simulink model "MotorXploer"  (R2025a)
settings: Solver=FixedStepAuto  StartTime=0.0  StopTime=inf  FixedStep=0.001  RelTol=1e-3
undefined symbols (not defined in the file): Blocking, LF, Non
libraries: amg_usbconverter_n_connect_lib x3, dspstat3 x2, simulink x2, dspfdesign x1, waijung_addon_module x1
settings Model: Creator=beamk  LastModifiedBy=nitic

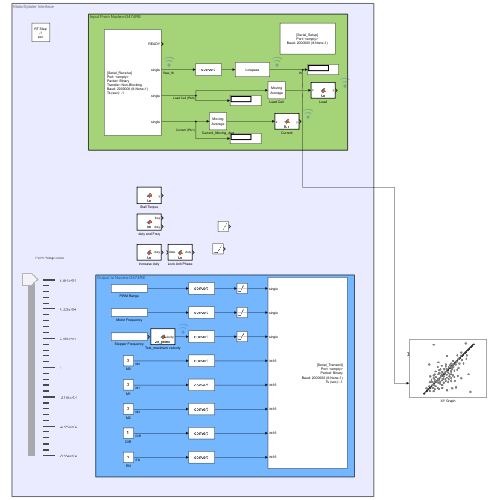
[thumbnail: Simulink's stored preview of the top-level diagram]
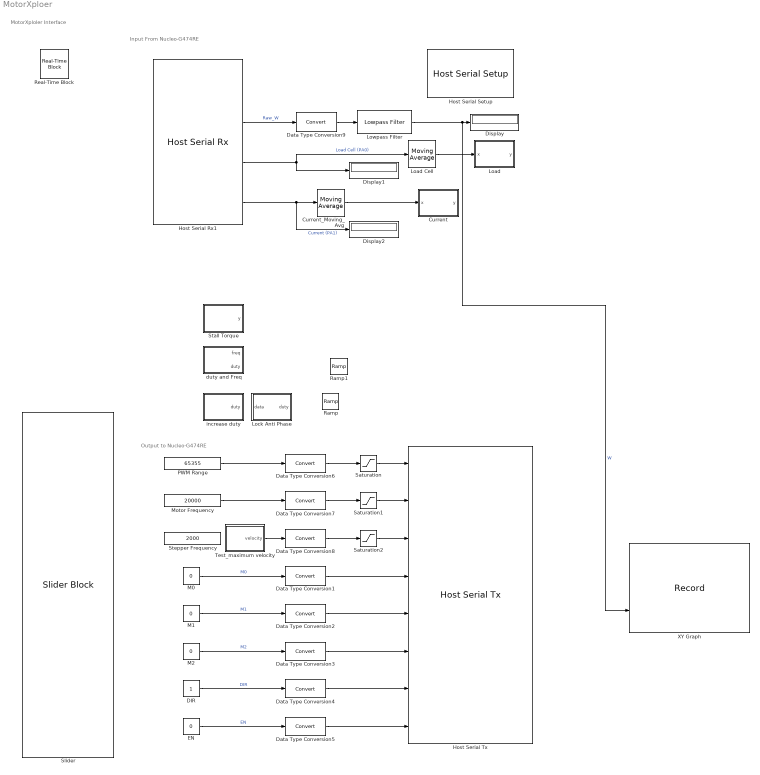
== system MotorXploer ==
  note: Output to Nucleo-G474RE
  note: Input From Nucleo-G474RE
  note: MotorXploler Interface
  Current : MATLAB Function  TreatAsAtomicUnit=on
  Current_Moving_Avg : dspstat3/Moving Average  Method=Sliding window  ForgettingFactorPort=off  SpecifyWindowLength=on  WindowLength=100  OverlapLength=99  AllowArbitraryInputLength=off  ForgettingFactor=0.9  SimulateUsing=Interpreted execution
  DIR : Constant
  Data Type Conversion{1..9} (9 alike) : DataTypeConversion  SaturateOnIntegerOverflow=off  RndMeth=Floor
  Display : Display
  Display1 : Display
  Display2 : Display
  EN : Constant  Value=0
  Host Serial Rx1 : amg_usbconverter_n_connect_lib/Host Serial Rx  conf=rx  port=<auto>  baudrate=2000000  databits=8  parity=None  stopbit=1  flowcontrol=None  transfer=Non-Blocking  timeout=5  packetmode=Binary  enableinitialvalues=off  initialvalues=[]  binheader='25'  binterminator='4E'  porttype_double=0  porttype_single=3  porttype_int8=0  porttype_uint8=0  porttype_int16=0  porttype_uint16=0  porttype_int32=0  porttype_uint32=0  asciiformat='%f,%f,%d,%d'  rx_asciiterminator="LF (0x0A - \"\\n\")"  tx_asciiterminator="CRLF (0x0D 0x0A - \"\\r\\n\")"  sampletime=-1  enablecustomportlabel=off  cinputportlabel=0  coutputportlabel=A  portpinstr=0  blockid=HostSerialRx1  inputporttype=[]  inputportwidth=[]  inputportlabel={}  outputporttype=[3 1 1 1]  outputportwidth=[1 1 1 1]  outputportlabel={'READY','single','single','single'}  compat=0  optionstring=[]  autoport='<empty>'
  Host Serial Setup : amg_usbconverter_n_connect_lib/Host Serial Setup  conf=setup  port=<auto>  baudrate=2000000  databits=8  parity=None  stopbit=1  flowcontrol=None  transfer=Blocking  timeout=2  packetmode=Binary  initialvalues=[]  binheader='7E 7E'  binterminator='03 03'  porttype_double=0  porttype_single=1  porttype_int8=0  porttype_uint8=0  porttype_int16=0  porttype_uint16=0  porttype_int32=0  porttype_uint32=2  asciiformat='%d %u %x'  rx_asciiterminator="CRLF (0x0D 0x0A - \"\\r\\n\")"  tx_asciiterminator="CRLF (0x0D 0x0A - \"\\r\\n\")"  sampletime=-1  enablecustomportlabel=off  cinputportlabel=0  coutputportlabel=A  portpinstr=0  blockid=HostSerialSetup  inputporttype=[]  inputportwidth=[]  inputportlabel={}  outputporttype=[]  outputportwidth=[]  outputportlabel={}  compat=0  optionstring=[]  autoport='<empty>'
  Host Serial Tx : amg_usbconverter_n_connect_lib/Host Serial Tx  conf=tx  port=<auto>  baudrate=2000000  databits=8  parity=None  stopbit=1  flowcontrol=None  transfer=Blocking  timeout=2  packetmode=Binary  initialvalues=[]  binheader='25'  binterminator='4E'  porttype_double=0  porttype_single=3  porttype_int8=0  porttype_uint8=0  porttype_int16=5  porttype_uint16=0  porttype_int32=0  porttype_uint32=0  asciiformat='%d,%f'  rx_asciiterminator="CRLF (0x0D 0x0A - \"\\r\\n\")"  tx_asciiterminator="CRLF (0x0D 0x0A - \"\\r\\n\")"  sampletime=-1  enablecustomportlabel=off  cinputportlabel=0  coutputportlabel=A  portpinstr=0  blockid=HostSerialTx  inputporttype=[1 1 1 4 4 4 4 4]  inputportwidth=[1 1 1 1 1 1 1 1]  inputportlabel={'single','single','single','int16','int16','int16','int16','int16'}  outputporttype=[]  outputportwidth=[]  outputportlabel={}  compat=0  optionstring=[]  autoport='<empty>'
      settings: SourceProductName=aMG USB Converter N
  Load : MATLAB Function  TreatAsAtomicUnit=on
  Load Cell : dspstat3/Moving Average  Method=Sliding window  ForgettingFactorPort=off  SpecifyWindowLength=on  WindowLength=500  OverlapLength=499  AllowArbitraryInputLength=off  ForgettingFactor=0.9  SimulateUsing=Interpreted execution
  Lock Anti Phase : MATLAB Function  TreatAsAtomicUnit=on
  Lowpass Filter : dspfdesign/Lowpass Filter  FilterType=FIR  DesignForMinimumOrder=on  FilterOrder=50  PassbandFrequency=7.5  StopbandFrequency=15  PassbandRipple=0.1  StopbandAttenuation=80  SampleRateMode=Specify on dialog  SampleRate=1000  SimulateUsing=Interpreted execution  roundingMode=Floor  coeffsDataTypeStr=fixdt(1,16)
  M0 : Constant  Value=0
  M1 : Constant  Value=0
  M2 : Constant  Value=0
  Motor Frequency : Constant  Value=20000  OutDataTypeStr=single
  PWM Range : Constant  Value=65355  OutDataTypeStr=single
  Ramp : simulink/Sources/Ramp  slope=65535/20  start=2  InitialOutput=0
  Ramp1 : simulink/Sources/Ramp  slope=320000/30  start=2  InitialOutput=0
  Real-Time Block : waijung_addon_module/Real-Time Block  Priority=0  setting=Default  sampletime=-1
      settings: SourceProductName=Misc
  Saturation : Saturate  UpperLimit=65535  LowerLimit=-65535
  Saturation1 : Saturate  UpperLimit=20000  LowerLimit=0
  Saturation2 : Saturate  UpperLimit=inf  LowerLimit=0
  Slider : SliderBlock  ScaleMin=-65535  ScaleMax=65535
  Stall Torque : MATLAB Function  TreatAsAtomicUnit=on
  Stepper Frequency : Constant  Value=2000  OutDataTypeStr=single
  Test_maximum velocity : MATLAB Function  TreatAsAtomicUnit=on
  XY Graph : Record  NumPorts=2.0  FileSettingsInternal="{\"entries\":[{\"content\":{\"excelSettings\":{\"content\":{},\"type\":\"Streamout.ExcelSettings\"},\"parquetSettings\":{\"content\":{},\"type\":\"Streamout.ParquetSettings\"}},\"type\":\"Streamout.FileSettingStorage\",\"uuid\":\"\"}],\"packageUris\":[\"http:\\/\\/schema.mathworks.com\\/mf0\\/streamout_blocks\\/R2020a\"],\"version\":\"1.0\"}"  FrameSettings=[0, 0]  Layout=[1 1]  SignalsInternal="{\"entries\":[{\"content\":{\"signals\":[{\"content\":{\"blockPath\":[],\"dimensions\":[1],\"domain\":\"\",\"lineColor\":\"#a2142f\",\"plots\":[ 1 ],\"port\":1,\"signalID\":1},\"type\":\"RecordBlkView.Signal\",\"uuid\":\"\"},{\"content\":{\"blockPath\":[],\"dimensions\":[1,1],\"domain\":\"\",\"lineColor\":\"#139fff\",\"plots\":[ 1 ],\"port\":2,\"signalID\":2,\"signalName\":\"W\"},\"type\":\"RecordBlkView.Signal\",\"uuid\":\"\"}]},\"type\":\"RecordBlkView.InputSignals\",\"uuid\":\"\"}],\"packageUris\":[\"http:\\/\\/schema.mathworks.com\\/mf0\\/streamout_blocks\\/R2020a\"],\"version\":\"1.0\"}"  VisualizationBindings="{\"xyplotplugin\":{\"info\":[{\"series\":[{\"bindingParametersList\":[{\"parameter\":\"X-Axis\",\"signalID\":1,\"signalName\":\"XY Graph:1\"},{\"parameter\":\"Y-Axis\",\"signalID\":2,\"signalName\":\"W\"}],\"seriesID\":0}],\"subplotID\":1}]}}"  CompatibilityTag=XY
  duty and Freq : MATLAB Function  TreatAsAtomicUnit=on
  increase duty : MATLAB Function  TreatAsAtomicUnit=on
  wires:
  Host Serial Rx1/3 -> Load Cell/1, Display1/1  "Load Cell (PA0)"
  M0/1 -> Data Type Conversion1/1  "M0"
  EN/1 -> Data Type Conversion5/1  "EN"
  DIR/1 -> Data Type Conversion4/1  "DIR"
  M1/1 -> Data Type Conversion2/1  "M1"
  M2/1 -> Data Type Conversion3/1  "M2"
  Data Type Conversion1/1 -> Host Serial Tx/4
  Data Type Conversion2/1 -> Host Serial Tx/5
  Data Type Conversion3/1 -> Host Serial Tx/6
  Data Type Conversion4/1 -> Host Serial Tx/7
  Data Type Conversion5/1 -> Host Serial Tx/8
  Data Type Conversion6/1 -> Saturation/1
  Saturation/1 -> Host Serial Tx/1
  Data Type Conversion7/1 -> Saturation1/1
  Data Type Conversion8/1 -> Saturation2/1
  Saturation1/1 -> Host Serial Tx/2
  Saturation2/1 -> Host Serial Tx/3
  Host Serial Rx1/4 -> Current_Moving_Avg/1, Display2/1  "Current (PA1)"
  Current_Moving_Avg/1 -> Current/1(x)
  Load Cell/1 -> Load/1(x)
  Lowpass Filter/1 -> XY Graph/2, Display/1  "W"
  Motor Frequency/1 -> Data Type Conversion7/1
  Data Type Conversion9/1 -> Lowpass Filter/1
  Host Serial Rx1/2 -> Data Type Conversion9/1  "Raw_W"
  PWM Range/1 -> Data Type Conversion6/1
  Test_maximum velocity/1(velocity) -> Data Type Conversion8/1

== matlab function MotorXploer/Current ==
  data: x input; y output
function y = fcn(x)
y= -0.0148*x+31.4+0.2;

== matlab function MotorXploer/Load ==
  data: x input; y output
function y = fcn(x)
y= 0.2556*x-163.04-10;

== matlab function MotorXploer/Stall Torque ==
  data: y output
function y = fcn()
% --- 1. ตั้งค่า Sample Time (สำคัญมาก!) ---
% ให้ใส่ค่า Fixed-step size ของโมเดลคุณที่นี่
Ts = 0.001;  % <--- !!! ต้องเปลี่ยนค่านี้นะครับ !!!

% --- 2. คำนวณจำนวน Step ที่ต้องการสำหรับแต่ละสถานะ ---
STEPS_1 = round(5.0 / Ts); % 5 วินาที
STEPS_2 = round(0.5 / Ts); % 2 วินาที
STEPS_3 = round(2.0 / Ts); % 2 วินาที

val = -65536; % 2^16

% --- 3. สร้างตัวแปรเก็บสถานะ (State) และตัวนับ (Counter) ---
persistent state;
persistent counter;
persistent y_out;  % <--- เพิ่มตัวแปรนี้เข้ามา

% --- 4. ตรวจสอบค่าเริ่มต้น (ถ้ายังไม่เคยรัน) ---
if isempty(state)
    % เริ่มต้นที่สถานะ 1
    state = 1;
    counter = 0;
    y_out = val;   % <--- กำหนดค่าเริ่มต้นให้ y_out
end

% --- 5. ตรรกะ State Machine ---
switch state
    case 1  % --- สถานะที่ 1 ---
        y_out = val; % อัปเดต y_out
        counter = counter + 1;
        % ตรวจสอบว่าครบ 5 วิ หรือยัง
        if counter >= STEPS_1
            state = 2;      % ไปสถานะ 2
            counter = 0;    % รีเซ็ตตัวนับ
        end
        
    case 2  % --- สถานะที่ 2 ---
        y_out = -val; % อัปเดต y_out
        counter = counter + 1;
        % ตรวจสอบว่าครบ 2 วิ หรือยัง
        if counter >= STEPS_2
            state = 3;      % ไปสถานะ 3
            counter = 0;    % รีเซ็ตตัวนับ
        end
        
    case 3  % --- สถานะที่ 3 ---
        y_out = 0; % อัปเดต y_out
        counter = counter + 1;
        % ตรวจสอบว่าครบ 2 วิ หรือยัง
        if counter >= STEPS_3
            state = 1;      % วนกลับไปสถานะ 1
            counter = 0;    % รีเซ็ตตัวนับ
        end
end

% --- 6. ส่งค่าออก (รับประกันว่า y มีค่าเสมอ) ---
y = y_out; % <--- 'y' จะถูกกำหนดค่าในบรรทัดนี้เสมอ

== matlab function MotorXploer/duty and Freq ==
  data: freq output; duty output
function [freq, duty] = fcn()
% --- 1. ตั้งค่าพื้นฐาน ---
% *** สำคัญมาก: ตั้งค่า Ts ให้ตรงกับ Fixed-step size ของโมเดล ***
Ts = 0.01; % (เช่น 0.01, 0.001) ต้องตรงกับ Model Settings > Solver

% ค่าคงที่
FREQ_VAL = 5000;
DUTY_ON = 32768; % (2^16) * 0.5
DUTY_OFF = 0;
TOTAL_CYCLES = 10; % จำนวนรอบที่ต้องการวน

% --- 2. คำนวณจำนวน Step ที่ต้องนับ (อิงจาก Ts) ---
STEPS_ON = round(5.0 / Ts); % 5 วินาที
STEPS_OFF = round(2.0 / Ts); % 2 วินาที

% --- 3. สร้างตัวแปร persistent (ตัวแปรที่จำค่าตัวเองได้) ---
persistent state_duty;  % สถานะ (1=ON, 2=OFF, 3=DONE)
persistent count_step;  % ตัวนับ step ภายในสถานะ
persistent count_cycle; % ตัวนับรอบ (0 ถึง 9)

% ตัวแปรสำหรับ output (ป้องกัน error 'undefined')
persistent freq_out;
persistent duty_out;

% --- 4. Initialization (ทำงานครั้งเดียวตอนเริ่ม Simulation) ---
if isempty(state_duty)
    % กำหนดค่าเริ่มต้นทั้งหมด
    state_duty = 1;     % เริ่มที่สถานะ ON
    count_step = 0;     % เริ่มที่ step ที่ 0
    count_cycle = 0;    % เริ่มที่รอบที่ 0
    
    % กำหนดค่า output เริ่มต้น
    freq_out = FREQ_VAL;
    duty_out = DUTY_ON;
end

% --- 5. State Machine หลัก ---
switch state_duty
    case 1  % --- สถานะ ON (5 วินาที) ---
        freq_out = FREQ_VAL;
        duty_out = DUTY_ON;
        
        count_step = count_step + 1;
        % ตรวจสอบว่าครบ 5 วิ หรือยัง
        if count_step >= STEPS_ON
            state_duty = 2;      % เปลี่ยนไปสถานะ OFF
            count_step = 0;    % รีเซ็ตตัวนับ step
        end
        
    case 2  % --- สถานะ OFF (2 วินาที) ---
        freq_out = FREQ_VAL;
        duty_out = DUTY_OFF;
        
        count_step = count_step + 1;
        % ตรวจสอบว่าครบ 2 วิ หรือยัง
        if count_step >= STEPS_OFF
            count_cycle = count_cycle + 1; % เพิ่มตัวนับรอบ (จบ 1 รอบ)
            
            % ตรวจสอบว่าครบ 10 รอบหรือยัง
            if count_cycle < TOTAL_CYCLES
                state_duty = 1;      % ยังไม่ครบ -> กลับไปสถานะ ON
            else
                state_duty = 3;      % ครบ 10 รอบแล้ว -> ไปสถานะ DONE
            end
            count_step = 0;    % รีเซ็ตตัวนับ step
        end
        
    case 3 % --- สถานะ DONE (หลังจากครบ 10 รอบ) ---
        % ค้างค่าสุดท้ายไว้ (freq=200, duty=0)
        % ไม่ต้องทำอะไร ปล่อยให้ค่า freq_out, duty_out เป็นค่าเดิม
        freq_out = FREQ_VAL;
        duty_out = DUTY_OFF;
end

% --- 6. ส่งค่า Output ---
% (วิธีนี้รับประกันว่า freq และ duty มีค่าเสมอ)
freq = freq_out;
duty = duty_out;

== matlab function MotorXploer/increase duty ==
  data: duty output
function duty = fcn()
% --- 1. ตั้งค่าพื้นฐาน ---
% *** สำคัญมาก: ตั้งค่า Ts ให้ตรงกับ Fixed-step size ของโมเดล ***
Ts = 0.001; % (เช่น 0.01, 0.001) ต้องตรงกับ Model Settings > Solver

% ค่า Delay ที่ต้องการ
DELAY_TIME = 2.0; % Delay 2 วินาที

% ค่าการเปลี่ยนแปลง (เหมือนเดิม)
TIME_STEP = 0.2; % เพิ่มค่าทุกๆ 0.1 วินาที
DUTY_STEP = 65535/100;   % เพิ่มขึ้นทีละ 1
MAX_DUTY = 65535;  % ค่าสูงสุด
MIN_DUTY = 0;    % ค่าเริ่มต้น

% --- 2. คำนวณจำนวน Step ที่ต้องนับ (อิงจาก Ts) ---
STEPS_DELAY = round(DELAY_TIME / Ts); % จำนวน steps สำหรับ 2 วิ
STEPS_PER_INCREMENT = round(TIME_STEP / Ts); % จำนวน steps สำหรับ 0.1 วิ

% --- 3. สร้างตัวแปร persistent (ตัวแปรที่จำค่าตัวเองได้) ---
persistent state;       % 1=DELAY, 2=RAMPING, 3=DONE
persistent count_step;  % ตัวนับ step ภายในสถานะ
persistent duty_out;    % ค่า duty ที่จะส่งออกไป

% --- 4. Initialization (ทำงานครั้งเดียวตอนเริ่ม Simulation) ---
if isempty(state)
    % กำหนดค่าเริ่มต้นทั้งหมด
    state = 1; % <--- เริ่มที่ State 1 (DELAY)
    count_step = 0;
    duty_out = MIN_DUTY;
end

% --- 5. ตรรกะ State Machine ---
switch state
    case 1  % --- สถานะ 1: DELAY (2 วินาที) ---
        duty_out = MIN_DUTY; % คืนค่า 0 ตลอด
        count_step = count_step + 1;
        
        % ตรวจสอบว่าครบ 2 วิ หรือยัง
        if count_step >= STEPS_DELAY
            state = 2;       % ครบแล้ว, ไปสถานะ RAMPING
            count_step = 0;  % รีเซ็ตตัวนับสำหรับสถานะถัดไป
        end

    case 2  % --- สถานะ 2: RAMPING (เพิ่มค่า 0 -> 100) ---
        count_step = count_step + 1;
        
        % ตรวจสอบว่าครบ 0.1 วิ หรือยัง
        if count_step >= STEPS_PER_INCREMENT
            count_step = 0; % รีเซ็ตตัวนับสำหรับ 0.1 วิ ถัดไป
            
            % ตรวจสอบว่ายังไม่ถึง 100
            if duty_out < MAX_DUTY
                duty_out = duty_out + DUTY_STEP; % บวกเพิ่ม 1
            else
                duty_out = MAX_DUTY; % ถ้าถึง 100 แล้ว
                state = 3;       % ไปสถานะ DONE
            end
        end

    case 3  % --- สถานะ 3: DONE (ค้างค่า 100) ---
        % ไม่ต้องทำอะไร, duty_out จะค้างอยู่ที่ 100
        duty_out = MAX_DUTY;
end

% --- 6. ส่งค่า Output ---
duty = duty_out;

== matlab function MotorXploer/Lock Anti Phase ==
  data: duty output; data input
function duty = fcn(data)
% --- 1. ตั้งค่าพื้นฐาน ---
% *** สำคัญมาก: ตั้งค่า Ts ให้ตรงกับ Fixed-step size ของโมเดล ***
Ts = 0.001; % (เช่น 0.01, 0.001) ต้องตรงกับ Model Settings > Solver

% ค่า Delay ที่ต้องการ
DELAY_TIME = 2.0; % Delay 2 วินาที

% ค่าการเปลี่ยนแปลง (เหมือนเดิม)
TIME_STEP = 0.2; % เพิ่มค่าทุกๆ 0.1 วินาที
DUTY_STEP = -65535/100;   % เพิ่มขึ้นทีละ 1
MAX_DUTY = -65535;  % ค่าสูงสุด
MIN_DUTY = 0;    % ค่าเริ่มต้น

% --- 2. คำนวณจำนวน Step ที่ต้องนับ (อิงจาก Ts) ---
STEPS_DELAY = round(DELAY_TIME / Ts); % จำนวน steps สำหรับ 2 วิ
STEPS_PER_INCREMENT = round(TIME_STEP / Ts); % จำนวน steps สำหรับ 0.1 วิ

% --- 3. สร้างตัวแปร persistent (ตัวแปรที่จำค่าตัวเองได้) ---
persistent state;       % 1=DELAY, 2=RAMPING, 3=DONE
persistent count_step;  % ตัวนับ step ภายในสถานะ
persistent duty_out;    % ค่า duty ที่จะส่งออกไป

% --- 4. Initialization (ทำงานครั้งเดียวตอนเริ่ม Simulation) ---
if isempty(state)
    % กำหนดค่าเริ่มต้นทั้งหมด
    state = 1; % <--- เริ่มที่ State 1 (DELAY)
    count_step = 0;
    duty_out = MIN_DUTY;
end

% --- 5. ตรรกะ State Machine ---
switch state
    case 1  % --- สถานะ 1: DELAY (2 วินาที) ---
        duty_out = MIN_DUTY; % คืนค่า 0 ตลอด
        count_step = count_step + 1;
        
        % ตรวจสอบว่าครบ 2 วิ หรือยัง
        if count_step >= STEPS_DELAY
            state = 2;       % ครบแล้ว, ไปสถานะ RAMPING
            count_step = 0;  % รีเซ็ตตัวนับสำหรับสถานะถัดไป
        end

    case 2  % --- สถานะ 2: RAMPING (เพิ่มค่า 0 -> 100) ---
        count_step = count_step + 1;
        
        % ตรวจสอบว่าครบ 0.1 วิ หรือยัง
        if count_step >= STEPS_PER_INCREMENT
            count_step = 0; % รีเซ็ตตัวนับสำหรับ 0.1 วิ ถัดไป
            
            % ตรวจสอบว่ายังไม่ถึง 100
            if duty_out > MAX_DUTY
                duty_out = duty_out + DUTY_STEP; % บวกเพิ่ม 1
            else
                duty_out = MAX_DUTY; % ถ้าถึง 100 แล้ว
                state = 3;       % ไปสถานะ DONE
            end
        end

    case 3  % --- สถานะ 3: DONE (ค้างค่า 100) ---
        % ไม่ต้องทำอะไร, duty_out จะค้างอยู่ที่ 100
        duty_out = MAX_DUTY;
end

% --- 6. ส่งค่า Output ---
duty = duty_out;

== matlab function MotorXploer/Test_maximum velocity ==
  data: velocity output
function velocity = vel_profile()

%--- Parameters (ปรับได้ทั้งหมด) ---
Vmax = 3000;         % ความเร็วสูงสุด
acc_start = 10000;    % ค่าเร่งเริ่มต้น
acc_step = 10000;     % เพิ่มทีละเท่าไรในแต่ละรอบ
acc_end = 100000;     % ค่าเร่งสูงสุด
hold_time = 2;       % เวลาค้างที่ Vmax
rest_time = 2;       % เวลาพักหลัง deceleration
dt = 0.001;          % sample time

%--- Persistent states ---
persistent v t state acc

if isempty(v)
    v = 0;                  % initial speed
    t = 0;                  % internal timer
    state = 1;              % start at accelerate
    acc = acc_start;        % initial acceleration
end

%----------- STATE MACHINE -----------
switch state
    
    %=============== 1) ACCELERATION =================
    case 1
        v = v + acc * dt;
        
        if v >= Vmax
            v = Vmax;
            state = 2;   % go to hold at Vmax
            t = 0;
        end

    %=============== 2) HOLD AT Vmax =================
    case 2
        v = Vmax;
        t = t + dt;
        
        if t >= hold_time
            state = 3;   % go to deceleration
            t = 0;
        end

    %=============== 3) DECELERATION =================
    case 3
        v = v - acc * dt;
        
        if v <= 0
            v = 0;
            state = 4;   % go to rest
            t = 0;
        end

    %=============== 4) REST AT v = 0 =================
    case 4
        v = 0;
        t = t + dt;
        
        if t >= rest_time
            % prepare next loop
            acc = acc + acc_step;
            if acc > acc_end
                acc = acc_start;     % loop back
            end
            
            state = 1;
            t = 0;
        end
end

%---------------- OUTPUT ----------------
velocity = v;
